simulink model "PR_sim_bahn_dreieck_23a"  (R2023a)
settings: Solver=FixedStepAuto  StartTime=0.0  StopTime=Te  FixedStep=Ts  RelTol=1e-3  EnableMultiTasking=on
values from neighbouring files (symbols this model uses):
  s0 = .5    (= 0.5)    [PR_init_Bahn.m]
  Ts = 1e-3    (= 0.001)    [PR_init_Bahn.m]    (also in PR_init_PnP.m = 0.01)
settings Model: Creator=Hoebarth  LastModifiedBy=Flo
settings SolverCC: AlgebraicLoopSolver=TrustRegion
settings DataIOCC: LimitDataPoints=on  SaveFormat=Array  SignalLoggingSaveFormat=ModelDataLogs  ReturnWorkspaceOutputs=off
settings OptimizationCC: LifeSpan=inf
settings DebuggingCC: SaveWithParameterizedLinksMsg=none  UnderspecifiedInitializationDetection=Classic  MergeDetectMultiDrivingBlocksExec=none  SignalResolutionControl=TryResolveAllWithWarning  MultiTaskDSMMsg=warning  MultiTaskCondExecSysMsg=none  UnconnectedInputMsg=warning  UnconnectedOutputMsg=warning  UnconnectedLineMsg=warning  SFUnexpectedBacktrackingDiag=warning  SFNoUnconditionalDefaultTransitionDiag=warning  SFExecutionAtInitializationDiag=none  ArithmeticOperatorsInVariantConditions=warning
settings HardwareCC: ProdBitPerPointer=32  ProdBitPerSizeT=32  ProdBitPerPtrDiffT=32  ProdLargestAtomicFloat=None  ProdIntDivRoundTo=Undefined  ProdEndianess=Unspecified  ProdWordSize=32  ProdHWDeviceType=32-bit Generic  TargetUnknown=on
settings ModelReferenceCC: EnableRefExpFcnMdlSchedulingChecks=on  PropagateSignalLabelsOutOfModel=off
settings SFSimCC: SimUseLocalCustomCode=off  SimParseCustomCode=off  CustomCodeUndefinedFunction=UseInterfaceOnly
settings RTWCC: RTWUseLocalCustomCode=off
settings CodeAppCC: StateflowObjectComments=on
settings GRTTargetCC: TargetFcnLib=ansi_tfl_tmw.mat  TargetLangStandard=C89/C90 (ANSI)  CombineOutputUpdateFcns=off  GRTInterface=on
settings ConfigComp: CovMetricSettings=dw  CovSaveCumulativeToWorkspaceVar=on  CovSaveSingleToWorkspaceVar=on  CovExternalEMLEnable=off

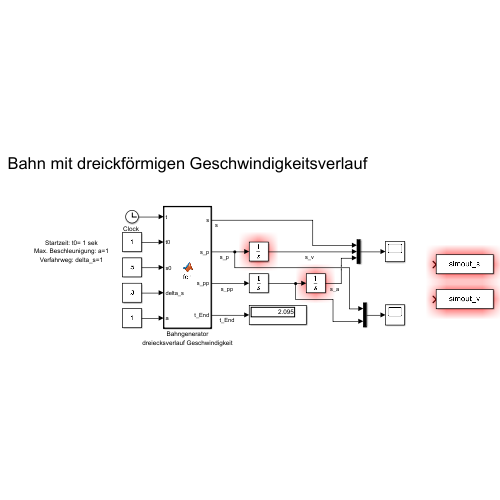
[thumbnail: Simulink's stored preview of the top-level diagram]
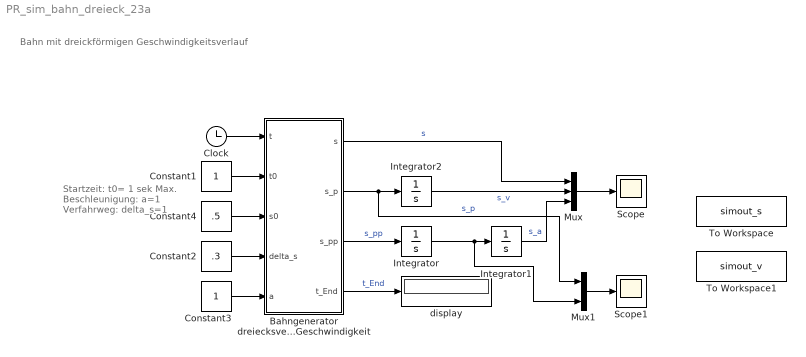
== system PR_sim_bahn_dreieck_23a ==
  note: Bahn mit dreickförmigen Geschwindigkeitsverlauf
  note: Startzeit: t0= 1 sek
      | Max. Beschleunigung: a=1
      | Verfahrweg: delta_s=1
  Bahngenerator dreiecksverlauf Geschwindigkeit : MATLAB Function  TreatAsAtomicUnit=on
  "Clock " : Clock
  Constant1 : Constant
  Constant2 : Constant  Value=.3
  Constant3 : Constant
  Constant4 : Constant  Value=.5
  Integrator : Integrator
  Integrator1 : Integrator  InitialCondition=s0
  Integrator2 : Integrator  InitialCondition=s0
  Mux : Mux  Inputs=3
  Mux1 : Mux  Inputs=2
  Scope : Scope
  Scope1 : Scope
  To Workspace : ToWorkspace  VariableName=simout_s  SaveFormat=Timeseries  SampleTime=Ts
  To Workspace1 : ToWorkspace  VariableName=simout_v  SaveFormat=Timeseries  SampleTime=Ts
  display : Display
  wires:
  "Clock "/1 -> Bahngenerator dreiecksverlauf Geschwindigkeit/1(t)
  Constant1/1 -> Bahngenerator dreiecksverlauf Geschwindigkeit/2(t0)
  Constant4/1 -> Bahngenerator dreiecksverlauf Geschwindigkeit/3(s0)
  Bahngenerator dreiecksverlauf Geschwindigkeit/4(t_End) -> display/1  "t_End"
  Bahngenerator dreiecksverlauf Geschwindigkeit/2(s_p) -> Mux1/1, Integrator2/1  "s_p"
  Bahngenerator dreiecksverlauf Geschwindigkeit/1(s) -> Mux/1  "s"
  Bahngenerator dreiecksverlauf Geschwindigkeit/3(s_pp) -> Integrator/1  "s_pp"
  Constant2/1 -> Bahngenerator dreiecksverlauf Geschwindigkeit/4(delta_s)
  Constant3/1 -> Bahngenerator dreiecksverlauf Geschwindigkeit/5(a)
  Integrator/1 -> Mux1/2, Integrator1/1
  Integrator1/1 -> Mux/3  "s_a"
  Integrator2/1 -> Mux/2  "s_v"
  Mux/1 -> Scope/1
  Mux1/1 -> Scope1/1

== matlab function PR_sim_bahn_dreieck_23a/Bahngenerator dreiecksverlauf Geschwindigkeit ==
  data: t input; s output; t0 input; s0 input; delta_s input; a input; s_p output; s_pp output; t_End output
function [s, s_p, s_pp, t_End] = fcn(t, t0, s0, delta_s, a)
%#codegen

% Mein erster Bahngenerator:
% in embeded Matlab functions kann mit gewoehnlichem m-Code (Matlab Code)
% gearbeitet werden.

% todo: Implementierung Bahngenerator

Ta = 2 * sqrt(abs(delta_s)/a);

if t < t0
    s = 0;
    s_p = 0;
    s_pp = 0;
elseif t < t0 + Ta/2
    s = a/2 * (-t0 + t)^2;
    s_p = a * (t - t0);
    s_pp = a;
elseif t < t0 + Ta
    s = a/2 * (-Ta^2 / 2 + 2*(t - t0)*Ta - (t - t0)^2);
    s_p = a * (t0 + Ta - t);
    s_pp = -a;
else
    s = a*Ta^2/4;
    s_p = 0;
    s_pp = 0;
end

s = s * sign(delta_s) + s0;
s_p = s_p * sign(delta_s);
s_pp = s_pp * sign(delta_s);

t_End = t0 + Ta;
